simulink model "L3_ocet_SystemSISOC"  (R2022b)
settings: Solver=ode45  StartTime=0.0  StopTime=tend  MaxStep=0.01  RelTol=1e-3  EnableMultiTasking=on
values from neighbouring files (symbols this model uses):
  sigma2e = 0.1    [L3_ocet_init.m]
  Tf = 2*Tp    (= 0.1)    [L3_ocet_init.m]
  Tp = 0.1    [L1_dzban_Init.m]    (also in L2_czolg_init.m; L3_ocet_init.m = 0.05)
libraries: simulink x1
settings Model: Creator=molsz  LastModifiedBy=molsz
settings SolverCC: AlgebraicLoopSolver=TrustRegion
settings DataIOCC: LimitDataPoints=on  SaveFormat=Array  SignalLoggingSaveFormat=ModelDataLogs  ReturnWorkspaceOutputs=off
settings OptimizationCC: InitFltsAndDblsToZero=on  LifeSpan=inf
settings DebuggingCC: SaveWithParameterizedLinksMsg=none  UnderspecifiedInitializationDetection=Classic  MergeDetectMultiDrivingBlocksExec=none  SignalResolutionControl=TryResolveAllWithWarning  SolverPrmCheckMsg=warning  MultiTaskDSMMsg=warning  MultiTaskCondExecSysMsg=none  FcnCallInpInsideContextMsg=warning  UnconnectedInputMsg=warning  UnconnectedOutputMsg=warning  UnconnectedLineMsg=warning  SFUnexpectedBacktrackingDiag=warning  SFNoUnconditionalDefaultTransitionDiag=warning  SFExecutionAtInitializationDiag=none  SFMachineParentedDataDiag=warning  ArithmeticOperatorsInVariantConditions=warning
settings HardwareCC: ProdBitPerPointer=32  ProdBitPerSizeT=32  ProdBitPerPtrDiffT=32  ProdLargestAtomicFloat=None  ProdIntDivRoundTo=Undefined  ProdEndianess=Unspecified  ProdWordSize=32  ProdHWDeviceType=32-bit Generic
settings ModelReferenceCC: PropagateSignalLabelsOutOfModel=off
settings CodeAppCC: StateflowObjectComments=on
settings GRTTargetCC: TargetFcnLib=ansi_tfl_tmw.mat  TargetLangStandard=C89/C90 (ANSI)  CombineOutputUpdateFcns=off  GRTInterface=on
settings ConfigComp: CovMetricSettings=dw  CovSaveCumulativeToWorkspaceVar=on  CovSaveSingleToWorkspaceVar=on

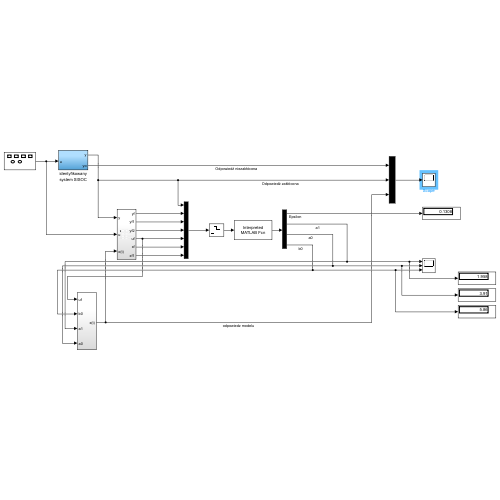
[thumbnail: Simulink's stored preview of the top-level diagram]
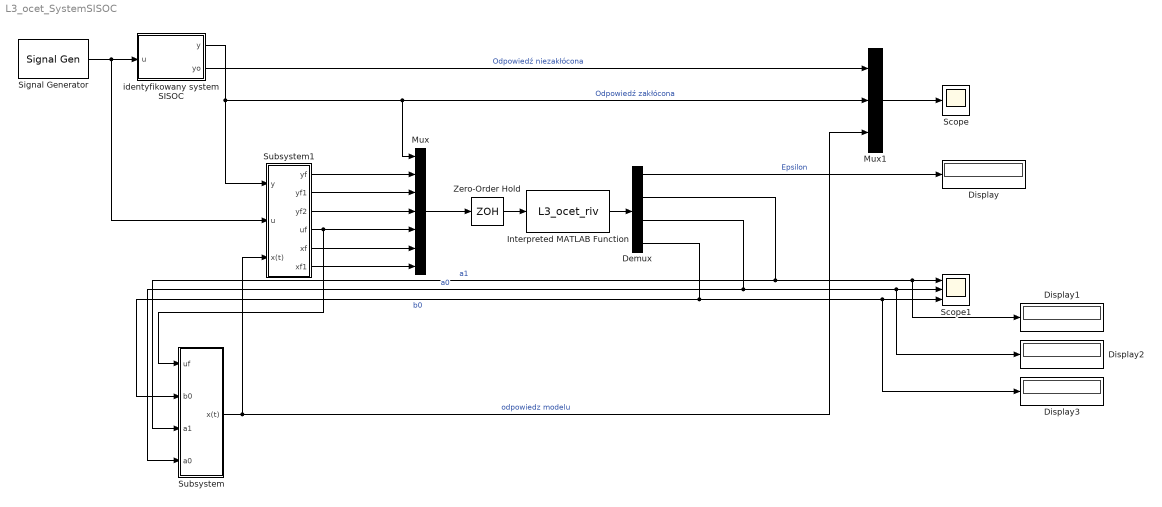
== system L3_ocet_SystemSISOC ==
  Demux : Demux
  Display{,1..3} (4 alike) : Display
  Interpreted MATLAB Function : MATLABFcn  MATLABFcn=L3_ocet_riv  OutputDimensions=4
  Mux : Mux  Inputs=7
  Mux1 : Mux  Inputs=3
  Scope : Scope
  Scope1 : Scope  NumInputPorts=3
  Signal Generator : SignalGenerator  WaveForm=square  Frequency=0.04
  Subsystem : Subsystem
  Subsystem1 : Subsystem
  Zero-Order Hold : ZeroOrderHold  SampleTime=Tp
  identyfikowany system SISOC : Subsystem
  wires:
  Signal Generator/1 -> Subsystem1/2(u), identyfikowany system SISOC/1(u)
  identyfikowany system SISOC/1(y) -> Subsystem1/1(y), Mux/1, Mux1/2  "Odpowiedź zakłócona"
  Subsystem1/4(uf) -> Subsystem/1(uf), Mux/5
  Mux/1 -> Zero-Order Hold/1
  Zero-Order Hold/1 -> Interpreted MATLAB Function/1
  Interpreted MATLAB Function/1 -> Demux/1
  Demux/2 -> Display1/1, Scope1/1, Subsystem/3(a1)  "a1"
  Demux/3 -> Display2/1, Scope1/2, Subsystem/4(a0)  "a0"
  Demux/4 -> Display3/1, Scope1/3, Subsystem/2("b0 ")  "b0"
  Subsystem/1(x(t)) -> Mux1/3, Subsystem1/3(x(t))  "odpowiedz modelu"
  identyfikowany system SISOC/2(yo) -> Mux1/1  "Odpowiedź niezakłócona"
  Mux1/1 -> Scope/1
  Demux/1 -> Display/1  "Epsilon"
  Subsystem1/1(yf) -> Mux/2
  Subsystem1/2(yf1) -> Mux/3
  Subsystem1/3(yf2) -> Mux/4
  Subsystem1/5(xf) -> Mux/6
  Subsystem1/6(xf1) -> Mux/7

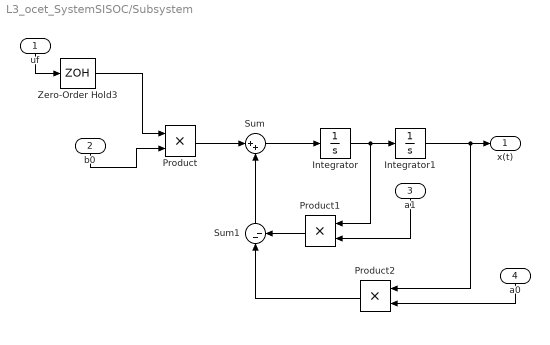
== system L3_ocet_SystemSISOC/Subsystem ==
  uf : Inport
  "b0 " : Inport  Port=2
  a1 : Inport  Port=3
  a0 : Inport  Port=4
  Integrator : Integrator
  Integrator1 : Integrator
  Product : Product  RndMeth=Zero  SampleTime=Tp
  Product1 : Product  RndMeth=Zero  SampleTime=Tp
  Product2 : Product  RndMeth=Zero  SampleTime=Tp
  Sum : Sum  Inputs=|++  SampleTime=Tp
  Sum1 : Sum  Inputs=|--  SampleTime=Tp
  Zero-Order Hold3 : ZeroOrderHold  SampleTime=Tp
  x(t) : Outport  VectorParamsAs1DForOutWhenUnconnected=off
  wires:
  Product/1 -> Sum/1
  Sum/1 -> Integrator/1
  Integrator/1 -> Integrator1/1, Product1/1
  Integrator1/1 -> x(t)/1, Product2/1
  Sum1/1 -> Sum/2
  Product1/1 -> Sum1/2
  Product2/1 -> Sum1/1
  a0/1 -> Product2/2
  uf/1 -> Zero-Order Hold3/1
  "b0 "/1 -> Product/2
  a1/1 -> Product1/2
  Zero-Order Hold3/1 -> Product/1

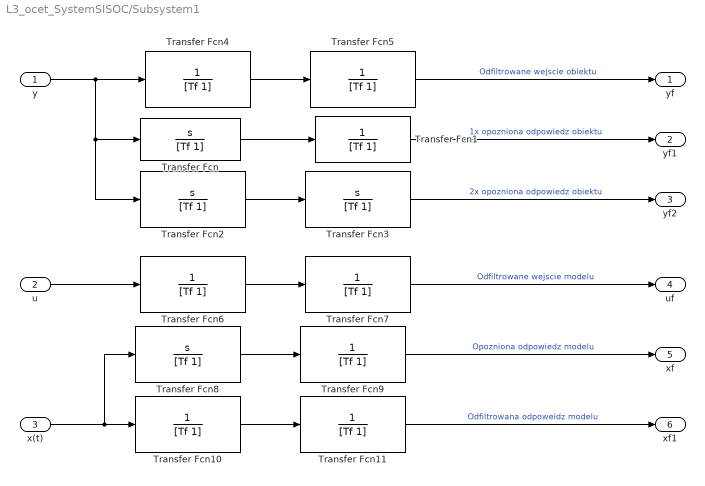
== system L3_ocet_SystemSISOC/Subsystem1 ==
  y : Inport
  u : Inport  Port=2
  x(t) : Inport  Port=3
  Transfer Fcn{,2..3,8} (4 alike) : TransferFcn  Numerator=[1 0]  Denominator=[Tf 1]
  Transfer Fcn{1,4..7,9..11} (8 alike) : TransferFcn  Denominator=[Tf 1]
  yf : Outport
  yf1 : Outport  Port=2
  yf2 : Outport  Port=3
  uf : Outport  Port=4
  xf : Outport  Port=5
  xf1 : Outport  Port=6
  wires:
  Transfer Fcn5/1 -> yf/1  "Odfiltrowane wejscie obiektu"
  y/1 -> Transfer Fcn/1, Transfer Fcn2/1, Transfer Fcn4/1
  Transfer Fcn6/1 -> Transfer Fcn7/1
  Transfer Fcn8/1 -> Transfer Fcn9/1
  Transfer Fcn10/1 -> Transfer Fcn11/1
  Transfer Fcn2/1 -> Transfer Fcn3/1
  Transfer Fcn/1 -> Transfer Fcn1/1
  Transfer Fcn11/1 -> xf1/1  "Odfiltrowana odpoweidz modelu"
  Transfer Fcn4/1 -> Transfer Fcn5/1
  Transfer Fcn9/1 -> xf/1  "Opozniona odpowiedz modelu"
  Transfer Fcn1/1 -> yf1/1  "1x opozniona odpowiedz obiektu"
  Transfer Fcn7/1 -> uf/1  "Odfiltrowane wejscie modelu"
  Transfer Fcn3/1 -> yf2/1  "2x opozniona odpowiedz obiektu"
  u/1 -> Transfer Fcn6/1
  x(t)/1 -> Transfer Fcn8/1, Transfer Fcn10/1

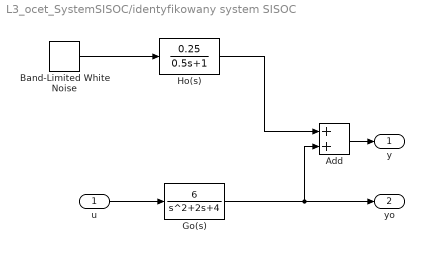
== system L3_ocet_SystemSISOC/identyfikowany system SISOC ==
  u : Inport
  Add : Sum
  Band-Limited White Noise : simulink/Sources/Band-Limited White Noise  Cov=[sigma2e]  Ts=Tp*0.1  seed=[2941]
  Go(s) : TransferFcn  Numerator=[6]  Denominator=[1 2 4]
  Ho(s) : TransferFcn  Numerator=[0.25]  Denominator=[0.5 1]
  y : Outport
  yo : Outport  Port=2
  wires:
  Band-Limited White Noise/1 -> Ho(s)/1
  Ho(s)/1 -> Add/1
  Go(s)/1 -> Add/2, yo/1
  Add/1 -> y/1
  u/1 -> Go(s)/1
